simulink model "Final_UKF_2018b"  (R2021a)
settings: Solver=ode4  StartTime=0.0  StopTime=200  FixedStep=1e-4  RelTol=1e-3
libraries: commchan3 x2
settings Model: Creator=12406  LastModifiedBy=aryal
settings SolverCC: AlgebraicLoopSolver=TrustRegion
settings DebuggingCC: ArithmeticOperatorsInVariantConditions=warning
settings SFSimCC: CustomCodeUndefinedFunction=UseInterfaceOnly

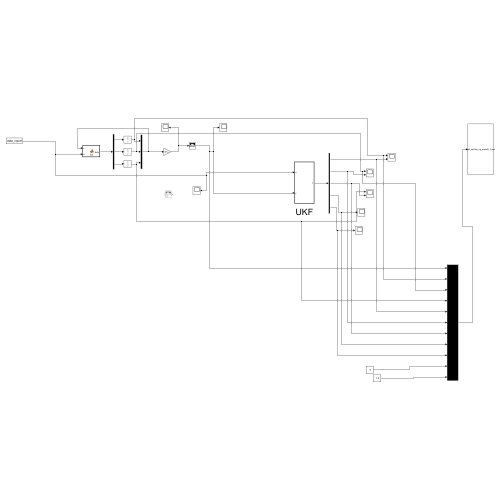
[thumbnail: Simulink's stored preview of the top-level diagram]
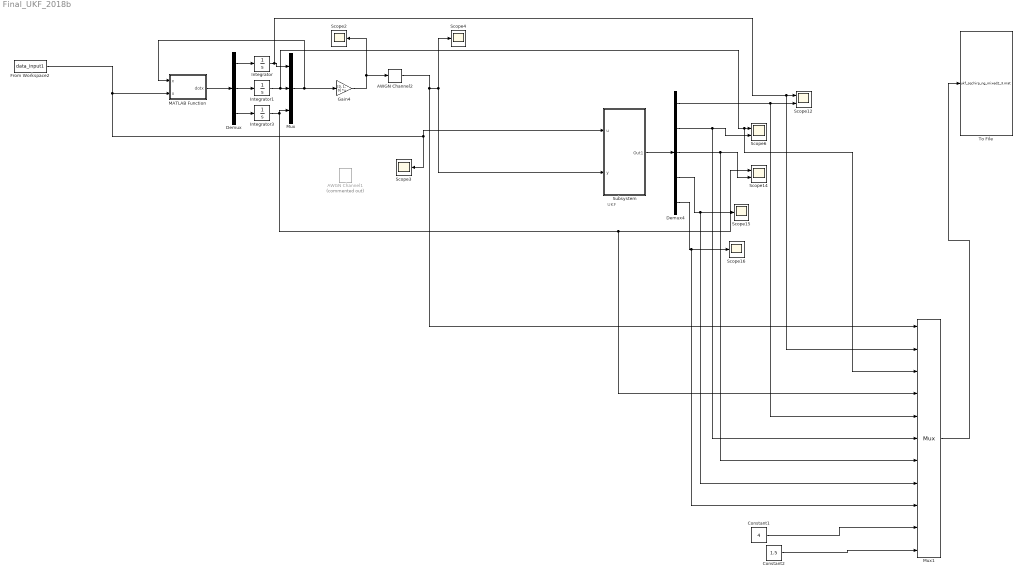
== system Final_UKF_2018b ==
  note: UKF
  AWGN Channel1 : commchan3/AWGN Channel  Commented=on  InputProcessing=Columns as channels (frame based)  seed=65  noiseMode=Variance from mask  EbNodB=10  EsNodB=10  SNRdB=65  bitsPerSym=1  Ps=1  Tsym=1  variance=1e-6
  AWGN Channel2 : commchan3/AWGN Channel  InputProcessing=Columns as channels (frame based)  seed=65  noiseMode=Variance from mask  EbNodB=10  EsNodB=10  SNRdB=65  bitsPerSym=1  Ps=1  Tsym=1  variance=1e-6
  Constant1 : Constant  Value=4
  Constant2 : Constant  Value=1.5
  Demux : Demux  Outputs=3
  Demux4 : Demux  Outputs=5
  From Workspace2 : FromWorkspace  VariableName=data_input1  SampleTime=0.02
  Gain4 : Gain  Gain=[0, 1, 0]  Multiplication=Matrix(K*u)
  Integrator : Integrator
  Integrator1 : Integrator
  Integrator3 : Integrator
  MATLAB Function : MATLAB Function  TreatAsAtomicUnit=on
  Mux : Mux  Inputs=3
  Mux1 : Mux  Inputs=11
  Scope12 : Scope  NumInputPorts=2
  Scope14 : Scope  NumInputPorts=2
  Scope{2..4,15..16} (5 alike) : Scope
  Scope6 : Scope  NumInputPorts=2
  Subsystem : Subsystem  TreatAsAtomicUnit=on  SystemSampleTime=0.02
  To File : ToFile  Filename=ukf_sqchirp_ng_mixed2_3.mat  MatrixName=w  SampleTime=0.02
  wires:
  Demux/1 -> Integrator/1
  Gain4/1 -> AWGN Channel2/1, Scope2/1
  Integrator3/1 -> Mux1/4, Scope14/1, Mux/3
  Integrator1/1 -> Mux1/3, Scope6/1, Mux/2
  From Workspace2/1 -> Scope3/1, Subsystem/1(u), MATLAB Function/2(u)
  Demux/2 -> Integrator1/1
  Demux/3 -> Integrator3/1
  AWGN Channel2/1 -> Mux1/1, Subsystem/2(y), Scope4/1
  Mux/1 -> Gain4/1, MATLAB Function/1(x)
  MATLAB Function/1(dotx) -> Demux/1
  Integrator/1 -> Mux1/2, Scope12/1, Mux/1
  Demux4/1 -> Mux1/5, Scope12/2
  Demux4/5 -> Mux1/9, Scope16/1
  Demux4/4 -> Mux1/8, Scope15/1
  Demux4/3 -> Mux1/7, Scope14/2
  Demux4/2 -> Mux1/6, Scope6/2
  Subsystem/1(Out1) -> Demux4/1
  Mux1/1 -> To File/1
  Constant1/1 -> Mux1/10
  Constant2/1 -> Mux1/11

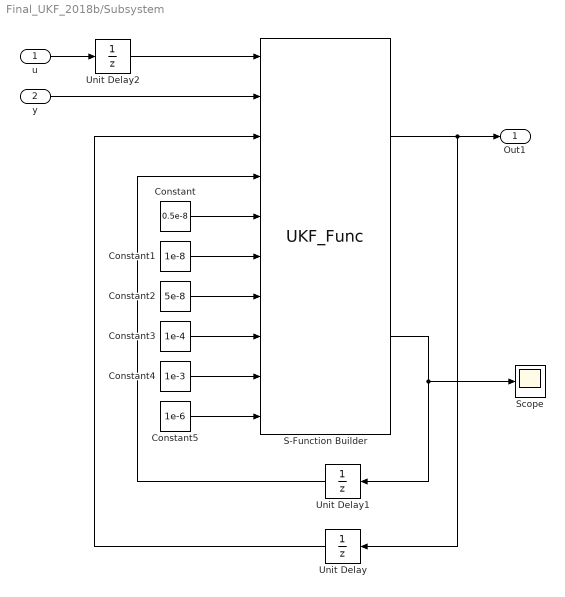
== system Final_UKF_2018b/Subsystem ==
  u : Inport
  y : Inport  Port=2
  Constant : Constant  Value=0.5e-8
  Constant1 : Constant  Value=1e-8
  Constant2 : Constant  Value=5e-8
  Constant3 : Constant  Value=1e-4
  Constant4 : Constant  Value=1e-3
  Constant5 : Constant  Value=1e-6
  S-Function Builder : S-Function  InitFcn=try, set_param(gcb,'FunctionName','UKF_Func'), end  FunctionName=UKF_Func  SFunctionModules=UKF_Func_wrapper UKF_Code UKF_Code_Call  SFunctionDeploymentMode=off  EnableBusSupport=off  mask(S-Function Builder){}
      mask help: Simulink:masks:SFunctionBuilder_MD
      mask init:
      | val = [[.9  0.75 0.75 1 1 .9 .9 1]',[1 1 0.75 0.75 .9 .9 1 .9]'];try , sys = get_param(gcb,'SfunBuilderFcnName');if isempty(sys), sys = get_param(gcb,'FunctionName'); end,catch, sys = get_param(gcb,'FunctionName'); end
      settings: CopyFcn=set_param(gcbh,'LinkStatus','none')  PreSaveFcn=try, set_param(gcb,'FunctionName','UKF_Func'), end  OpenFcn=sfunctionwizard(gcbh)
      mask Display: plot(val(:,1),val(:,2)),disp(sys),port_label('input',1,'u'),port_label('input',2,'y'),port_label('input',3,'xp'),port_label('input',4,'Pp'),port_label('input',5,'Q11'),port_label('input',6,'Q22'),port_label('input',7,'Q33'),port_label('input',8,'Q44'),port_label('input',9,'Q55'),port_label('input',10,'R'),port_label('output',1,'xhat'),port_label('output',2,'Phat')
  Scope : Scope
  Unit Delay : UnitDelay  InitialCondition=[0;0;0;2;2]  SampleTime=0.02  HasFrameUpgradeWarning=on
  Unit Delay1 : UnitDelay  InitialCondition=reshape(diag([10, 10, 10, 10, 10]), 25, 1)  SampleTime=0.02  HasFrameUpgradeWarning=on
  Unit Delay2 : UnitDelay  SampleTime=0.02  HasFrameUpgradeWarning=on
  Out1 : Outport
  wires:
  S-Function Builder/2 -> Scope/1, Unit Delay1/1
  Unit Delay/1 -> S-Function Builder/3
  y/1 -> S-Function Builder/2
  Unit Delay1/1 -> S-Function Builder/4
  S-Function Builder/1 -> Unit Delay/1, Out1/1
  u/1 -> Unit Delay2/1
  Unit Delay2/1 -> S-Function Builder/1
  Constant/1 -> S-Function Builder/5
  Constant1/1 -> S-Function Builder/6
  Constant2/1 -> S-Function Builder/7
  Constant3/1 -> S-Function Builder/8
  Constant4/1 -> S-Function Builder/9
  Constant5/1 -> S-Function Builder/10

== matlab function Final_UKF_2018b/MATLAB Function ==
  data: x input; u input; dotx output
function dotx  = fcn(x, u)
    D = 1.5;
    M = 4.0;
    Tg = 0.2;
    Rp = 0.05;
    Ki=2;
   dotx=zeros(3,1);
    x1 = x(1);
    x2 = x(2);
    x3 = x(3);
    dotx = [x2;x3;-Ki/(M*Tg)*x1-(D/(M*Tg)+1/(Rp*M*Tg))*x2-(D/M+1/Tg)*x3-1/(M*Tg)*u];
